simulink model "AmplitudVsPower"  (R2023a)
settings: Solver=FixedStepAuto  StartTime=0.0  StopTime=2  FixedStep=0.0001  RelTol=1e-3
settings Model: Creator=headl  LastModifiedBy=headl
settings DebuggingCC: UnconnectedInputMsg=warning  UnconnectedOutputMsg=warning  UnconnectedLineMsg=warning
settings ModelReferenceCC: EnableRefExpFcnMdlSchedulingChecks=on
settings RTWCC: DLArmComputeVersion=19.05

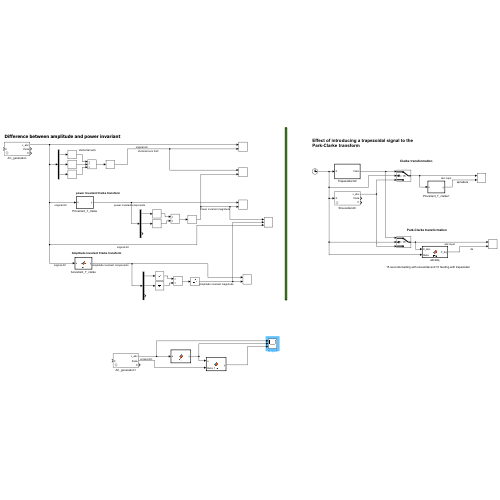
[thumbnail: Simulink's stored preview of the top-level diagram]
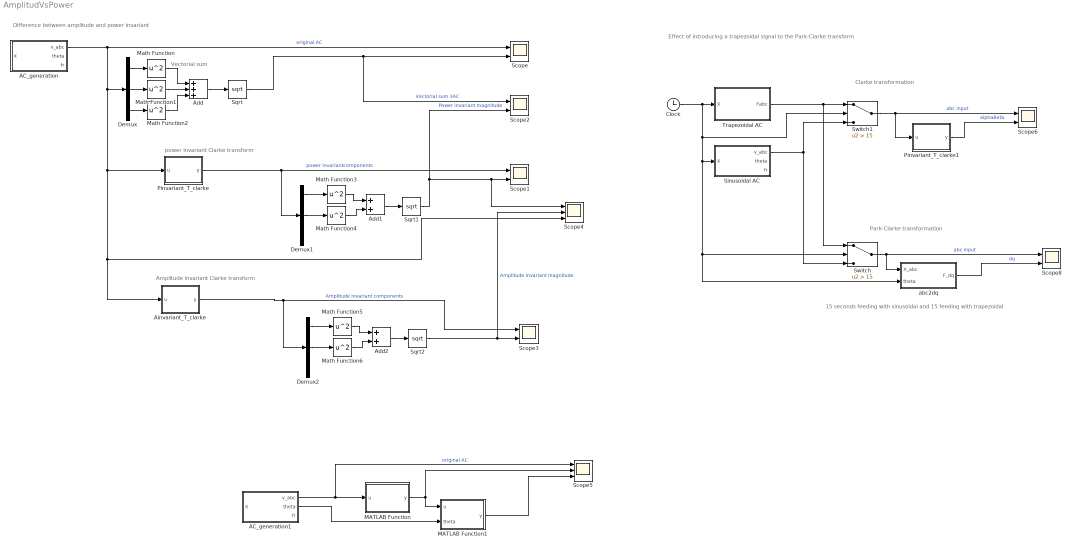
== system AmplitudVsPower ==
  note: 15 seconds feeding with sinusoidal and 15 feeding with trapezoidal
  note: Difference between amplitude and power invariant
  note: Effect of introducing a trapezoidal signal to the Park-Clarke transform
  note: Park-Clarke transformation
  note: Clarke transformation
  note: Amplitude invariant Clarke transform
  note: power invariant Clarke transform
  note: Vectorial sum
  AC_generation : Subsystem  mask{isSync=off, fr=1/(2*pi)}
      mask prompts: isSync "Synchronous"
  AC_generation1 : Subsystem  mask{isSync=off, fr=1}
      mask prompts: isSync "Synchronous"
  Add : Sum  Inputs=+++
  Add1 : Sum
  Add2 : Sum
  Ainvariant_T_clarke : MATLAB Function  TreatAsAtomicUnit=on
  Clock : Clock
  Demux : Demux  Outputs=3
  Demux1 : Demux  Outputs=3
  Demux2 : Demux  Outputs=3
  MATLAB Function : MATLAB Function  TreatAsAtomicUnit=on
  MATLAB Function1 : MATLAB Function  TreatAsAtomicUnit=on
  Math Function{,1..6} (7 alike) : Math  Operator=square
  Pinvariant_T_clarke : MATLAB Function  TreatAsAtomicUnit=on
  Pinvariant_T_clarke1 : MATLAB Function  TreatAsAtomicUnit=on
  Scope{,1..3,6,8} (6 alike) : Scope  NumInputPorts=2
  Scope4 : Scope  NumInputPorts=3
  Scope5 : Scope  NumInputPorts=3
  Sinusoidal AC : Subsystem  mask{isSync=on, fr=1/(2*pi)}
      mask prompts: isSync "Synchronous"
  Sqrt : Sqrt
  Sqrt1 : Sqrt
  Sqrt2 : Sqrt
  Switch : Switch  Criteria=u2 > Threshold  Threshold=15  SaturateOnIntegerOverflow=off  InputSameDT=off
  Switch1 : Switch  Criteria=u2 > Threshold  Threshold=15  SaturateOnIntegerOverflow=off  InputSameDT=off
  Trapezoidal AC : MATLAB Function  TreatAsAtomicUnit=on
  abc2dq : MATLAB Function  TreatAsAtomicUnit=on
  wires:
  AC_generation/1(v_abc) -> Scope4/3, Ainvariant_T_clarke/1(u), Pinvariant_T_clarke/1(u), Demux/1, Scope/1  "original AC"
  Demux/1 -> Math Function/1
  Math Function/1 -> Add/1
  Demux/2 -> Math Function1/1
  Demux/3 -> Math Function2/1
  Math Function1/1 -> Add/2
  Math Function2/1 -> Add/3
  Add/1 -> Sqrt/1
  Sqrt/1 -> Scope2/1, Scope/2  "Vectorial sum 3AC"
  Pinvariant_T_clarke/1(y) -> Demux1/1, Scope1/1  "power invariantcomponents"
  Demux1/1 -> Math Function3/1
  Demux1/2 -> Math Function4/1
  Math Function3/1 -> Add1/1
  Math Function4/1 -> Add1/2
  Add1/1 -> Sqrt1/1
  Sqrt1/1 -> Scope2/2, Scope4/1, Scope1/2  "Power invariant magnitude"
  Demux2/2 -> Math Function6/1
  Add2/1 -> Sqrt2/1
  Math Function5/1 -> Add2/1
  Demux2/1 -> Math Function5/1
  Math Function6/1 -> Add2/2
  Ainvariant_T_clarke/1(y) -> Scope3/1, Demux2/1  "Amplitude invariant components"
  Sqrt2/1 -> Scope4/2, Scope3/2  "Amplitude invariant magnitude"
  Clock/1 -> Switch/2, abc2dq/2(theta), Sinusoidal AC/1(X), Switch1/2, Trapezoidal AC/1(X)
  Trapezoidal AC/1(Fabc) -> Switch/1, Switch1/1
  Sinusoidal AC/1(v_abc) -> Switch1/3, Switch/3
  Switch/1 -> abc2dq/1(X_abc), Scope8/1  "abc input"
  abc2dq/1(F_dq) -> Scope8/2  "dq"
  Switch1/1 -> Scope6/1, Pinvariant_T_clarke1/1(u)  "abc input"
  Pinvariant_T_clarke1/1(y) -> Scope6/2  "alphaBeta"
  AC_generation1/1(v_abc) -> Scope5/1, MATLAB Function/1(u)  "original AC"
  MATLAB Function/1(y) -> MATLAB Function1/1(u), Scope5/2
  MATLAB Function1/1(y) -> Scope5/3
  AC_generation1/2(theta) -> MATLAB Function1/2(theta)

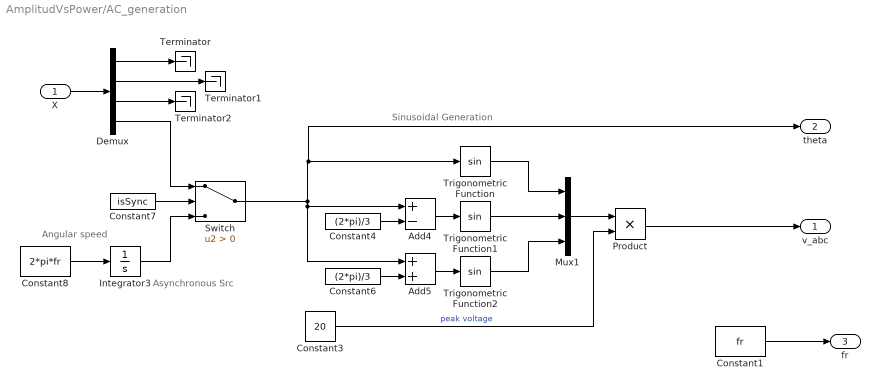
== system AmplitudVsPower/AC_generation ==
  note: Sinusoidal Generation
  note: Angular speed
  note: Asynchronous Src
  X : Inport
  Add4 : Sum  Inputs=+-
  Add5 : Sum
  Constant1 : Constant  Value=fr
  Constant3 : Constant  Value=20
  Constant4 : Constant  Value=(2*pi)/3
  Constant6 : Constant  Value=(2*pi)/3
  Constant7 : Constant  Value=isSync
  Constant8 : Constant  Value=2*pi*fr
  Demux : Demux
  Integrator3 : Integrator
  Mux1 : Mux  Inputs=3
  Product : Product
  Switch : Switch  Criteria=u2 > Threshold  SaturateOnIntegerOverflow=off  InputSameDT=off
  Terminator : Terminator
  Terminator1 : Terminator
  Terminator2 : Terminator
  Trigonometric Function : Trigonometry
  Trigonometric Function1 : Trigonometry
  Trigonometric Function2 : Trigonometry
  v_abc : Outport
  theta : Outport  Port=2
  fr : Outport  Port=3
  wires:
  Constant8/1 -> Integrator3/1
  Switch/1 -> Add5/1, Add4/1, theta/1, Trigonometric Function/1
  Constant3/1 -> Product/2  "peak voltage"
  Integrator3/1 -> Switch/3
  Demux/4 -> Switch/1
  Add5/1 -> Trigonometric Function2/1
  Trigonometric Function/1 -> Mux1/1
  Mux1/1 -> Product/1
  Trigonometric Function1/1 -> Mux1/2
  Trigonometric Function2/1 -> Mux1/3
  Constant7/1 -> Switch/2
  X/1 -> Demux/1
  Constant4/1 -> Add4/2
  Add4/1 -> Trigonometric Function1/1
  Constant6/1 -> Add5/2
  Product/1 -> v_abc/1
  Demux/1 -> Terminator/1
  Demux/3 -> Terminator2/1
  Demux/2 -> Terminator1/1
  Constant1/1 -> fr/1

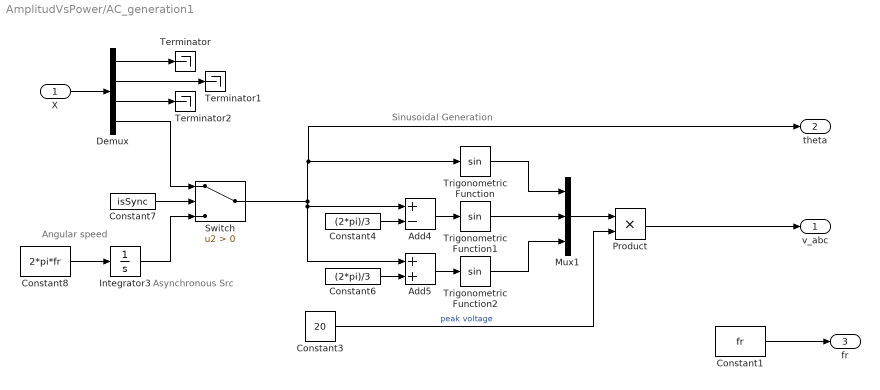
== system AmplitudVsPower/AC_generation1 ==
  note: Sinusoidal Generation
  note: Angular speed
  note: Asynchronous Src
  X : Inport
  Add4 : Sum  Inputs=+-
  Add5 : Sum
  Constant1 : Constant  Value=fr
  Constant3 : Constant  Value=20
  Constant4 : Constant  Value=(2*pi)/3
  Constant6 : Constant  Value=(2*pi)/3
  Constant7 : Constant  Value=isSync
  Constant8 : Constant  Value=2*pi*fr
  Demux : Demux
  Integrator3 : Integrator
  Mux1 : Mux  Inputs=3
  Product : Product
  Switch : Switch  Criteria=u2 > Threshold  SaturateOnIntegerOverflow=off  InputSameDT=off
  Terminator : Terminator
  Terminator1 : Terminator
  Terminator2 : Terminator
  Trigonometric Function : Trigonometry
  Trigonometric Function1 : Trigonometry
  Trigonometric Function2 : Trigonometry
  v_abc : Outport
  theta : Outport  Port=2
  fr : Outport  Port=3
  wires:
  Constant8/1 -> Integrator3/1
  Switch/1 -> Add5/1, Add4/1, theta/1, Trigonometric Function/1
  Constant3/1 -> Product/2  "peak voltage"
  Integrator3/1 -> Switch/3
  Demux/4 -> Switch/1
  Add5/1 -> Trigonometric Function2/1
  Trigonometric Function/1 -> Mux1/1
  Mux1/1 -> Product/1
  Trigonometric Function1/1 -> Mux1/2
  Trigonometric Function2/1 -> Mux1/3
  Constant7/1 -> Switch/2
  X/1 -> Demux/1
  Constant4/1 -> Add4/2
  Add4/1 -> Trigonometric Function1/1
  Constant6/1 -> Add5/2
  Product/1 -> v_abc/1
  Demux/1 -> Terminator/1
  Demux/3 -> Terminator2/1
  Demux/2 -> Terminator1/1
  Constant1/1 -> fr/1

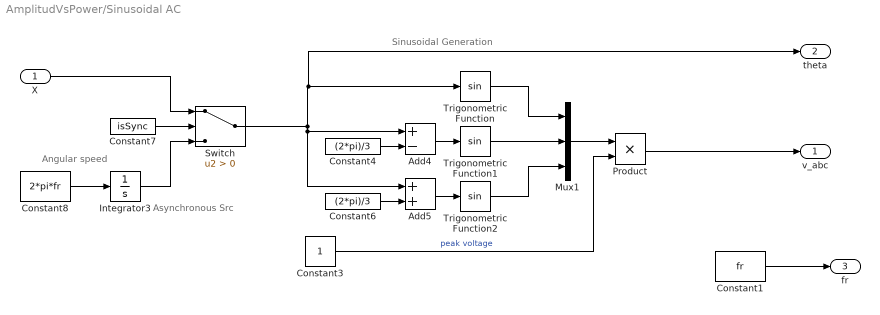
== system AmplitudVsPower/Sinusoidal AC ==
  note: Sinusoidal Generation
  note: Angular speed
  note: Asynchronous Src
  X : Inport
  Add4 : Sum  Inputs=+-
  Add5 : Sum
  Constant1 : Constant  Value=fr
  Constant3 : Constant
  Constant4 : Constant  Value=(2*pi)/3
  Constant6 : Constant  Value=(2*pi)/3
  Constant7 : Constant  Value=isSync
  Constant8 : Constant  Value=2*pi*fr
  Integrator3 : Integrator
  Mux1 : Mux  Inputs=3
  Product : Product
  Switch : Switch  Criteria=u2 > Threshold  SaturateOnIntegerOverflow=off  InputSameDT=off
  Trigonometric Function : Trigonometry
  Trigonometric Function1 : Trigonometry
  Trigonometric Function2 : Trigonometry
  v_abc : Outport
  theta : Outport  Port=2
  fr : Outport  Port=3
  wires:
  Constant8/1 -> Integrator3/1
  Switch/1 -> Add5/1, Add4/1, theta/1, Trigonometric Function/1
  Constant3/1 -> Product/2  "peak voltage"
  Integrator3/1 -> Switch/3
  X/1 -> Switch/1
  Add5/1 -> Trigonometric Function2/1
  Trigonometric Function/1 -> Mux1/1
  Mux1/1 -> Product/1
  Trigonometric Function1/1 -> Mux1/2
  Trigonometric Function2/1 -> Mux1/3
  Constant7/1 -> Switch/2
  Constant4/1 -> Add4/2
  Add4/1 -> Trigonometric Function1/1
  Constant6/1 -> Add5/2
  Product/1 -> v_abc/1
  Constant1/1 -> fr/1

== matlab function AmplitudVsPower/Ainvariant_T_clarke ==
  data: u input; y output
function y = fcn(u)


sC_Tst = 2/3*[ 1        -(1/2)        -(1/2) ; + ...
             -0       sqrt(3)/2    -sqrt(3)/2; + ...
            1/2          1/2           1/2];


y = sC_Tst*u;

== matlab function AmplitudVsPower/Pinvariant_T_clarke ==
  data: u input; y output
function y = fcn(u)


sC_T = sqrt(2/3)*[    1         -(1/2)        -(1/2);+ ...
                       0        sqrt(3)/2   -(sqrt(3)/2);+ ...
                  1/sqrt(2)    1/sqrt(2)    1/sqrt(2)];


y = sC_T*u;

== matlab function AmplitudVsPower/Pinvariant_T_clarke1 ==
  data: u input; y output
function y = fcn(u)


sC_T = sqrt(2/3)*[    1         -(1/2)        -(1/2);+ ...
                       0        sqrt(3)/2   -(sqrt(3)/2);+ ...
                  1/sqrt(2)    1/sqrt(2)    1/sqrt(2)];


y = sC_T*u;

== matlab function AmplitudVsPower/MATLAB Function ==
  data: u input; y output
function y = fcn(u)

sC_T = sqrt(2/3)*[    1         -(1/2)        -(1/2);
                      0        sqrt(3)/2   -(sqrt(3)/2);
                   1/sqrt(2)    1/sqrt(2)    1/sqrt(2)];

y = sC_T*u;

== matlab function AmplitudVsPower/MATLAB Function1 ==
  data: u input; y output; theta input
function y = fcn(u, theta)

sP_T = [  cos(theta)    sin(theta)   0;
          -sin(theta)   cos(theta)   0;
             0             0         1];
y = sP_T*u;

== matlab function AmplitudVsPower/abc2dq ==
  data: X_abc input; F_dq output; theta input
function F_dq = fcn(X_abc, theta)

% Park clarke transform eliminating the third element
PC_T = (sqrt(2)/2)*[sqrt(3)*cos(theta)  sin(theta)  -sin(theta) ; ...
                    -sqrt(3)*sin(theta)  cos(theta)  -cos(theta)];

F_dq = PC_T*X_abc;
                
end

== matlab function AmplitudVsPower/Trapezoidal AC ==
  data: X input; Fabc output
function Fabc = fcn(X)
Fabc = [0;0;0];
    theta = mod(X,2*pi);
    
    if (0<=theta)&&(theta<(pi/6))
        Fa = (6/pi)*theta;
    elseif ((pi/6)<=theta)&&(theta<(5*pi/6))
        Fa = 1;
    elseif ((5*pi/6<=theta))&&(theta<(7*pi/6))
        Fa = (6/pi)*(pi-theta);
    elseif ((7*pi/6)<=theta)&&(theta<(11*pi/6))
        Fa = -1;
    elseif ((11*pi/6)<=theta)&&(theta<(2*pi))
        Fa = (6/pi)*(theta-2*pi);
    else
        Fa = NaN;
    end
    
    if (0<=theta)&&(theta<(3*pi/6))
        Fb = -1;
    elseif ((3*pi/6)<=theta)&&(theta<(5*pi/6))
        Fb = (6/pi)*(theta-(2*pi)/3);
    elseif ((5*pi/6)<=theta)&&(theta<(9*pi/6))
        Fb = 1;
    elseif ((9*pi/6)<=theta)&&(theta<(11*pi/6))
        Fb = (6/pi)*(-theta+(5*pi)/3);
    elseif ((11*pi/6)<=theta)&&(theta<(2*pi))
        Fb = -1;
    else
        Fb = NaN;
    end
    
    if (0<=theta)&&(theta<(pi/6))
        Fc = 1;
    elseif ((pi/6)<=theta)&&(theta<(3*pi/6))
        Fc = (6/pi)*(pi/3-theta);
    elseif ((3*pi/6)<=theta)&&(theta<(7*pi/6))
        Fc = -1;
    elseif ((7*pi/6)<=theta)&&(theta<(9*pi/6))
        Fc = (6/pi)*(theta-(4*pi)/3);
    elseif ((9*pi/6)<=theta)&&(theta<(2*pi))
        Fc = 1;
    else
        Fc = NaN; 
    end
    
    Fabc = [Fa;Fb;Fc];
end
